simulink model "sim_model_ss"  (R2018b)
settings: Solver=VariableStepAuto  StartTime=0.0  StopTime=10.0  RelTol=1e-3
values from neighbouring files (symbols this model uses):
  A = J    [Main.m]
  B = [0;0;K6]    [Main.m]
  C1 = [1, 0, 0]    [Main.m]
  C2 = [0, 1, 0]    [Main.m]
  C3 = [0, 0, 1]    [Main.m]
  D = 0    [Main.m]
  u0 = er    [Main.m]
  x10 = 0.03    [Main.m]
  x20 = v0    (= 0)    [Main.m]
  x30 = I0    [Main.m]
settings Model: Creator=Eduardo  LastModifiedBy=ohara

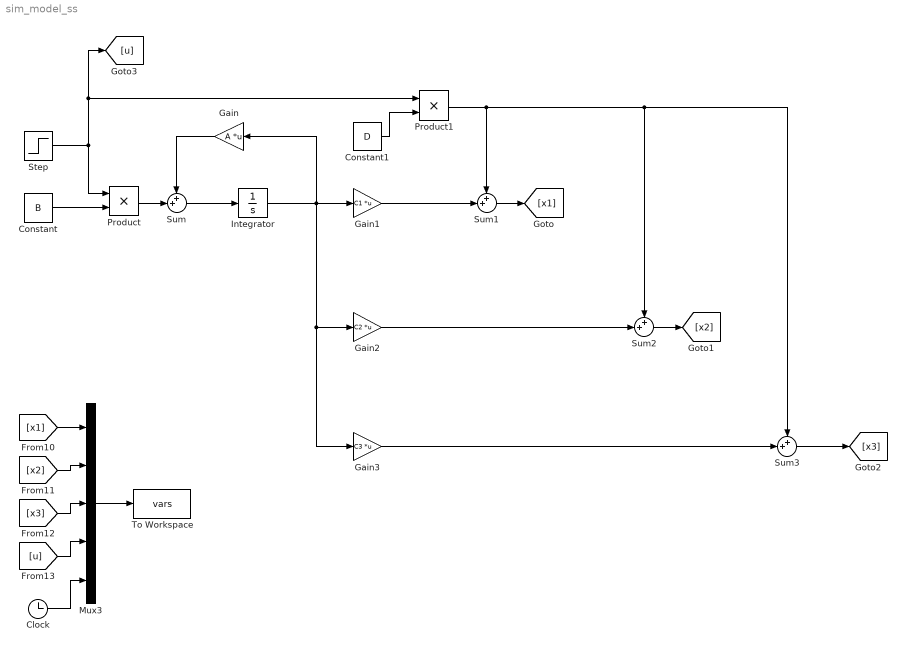
== system sim_model_ss ==
  Clock : Clock
  Constant : Constant  Value=B
  Constant1 : Constant  Value=D
  Gain : Gain  Gain=A  Multiplication=Matrix(K*u)
  Gain1 : Gain  Gain=C1  Multiplication=Matrix(K*u)
  Gain2 : Gain  Gain=C2  Multiplication=Matrix(K*u)
  Gain3 : Gain  Gain=C3  Multiplication=Matrix(K*u)
  Integrator : Integrator  InitialCondition=[x10;x20;x30]
  Mux3 : Mux  Inputs=5
  Product : Product
  Product1 : Product
  Step : Step  Time=0  Before=u0  After=u0  SampleTime=0
  Sum{,1..3} (4 alike) : Sum  Inputs=++|
  To Workspace : ToWorkspace  VariableName=vars  SaveFormat=Timeseries  SampleTime=-1
  wires:
  Sum/1 -> Integrator/1
  Product/1 -> Sum/2
  Constant/1 -> Product/2
  Step/1 -> Product/1, [u], Product1/1
  Gain/1 -> Sum/1
  Integrator/1 -> Gain2/1, Gain3/1, Gain1/1, Gain/1
  Gain1/1 -> Sum1/2
  Product1/1 -> Sum2/1, Sum3/1, Sum1/1
  Constant1/1 -> Product1/2
  Sum1/1 -> [x1]
  Gain2/1 -> Sum2/2
  Sum2/1 -> [x2]
  Gain3/1 -> Sum3/2
  Sum3/1 -> [x3]
  [x1] -> Mux3/1
  Clock/1 -> Mux3/5
  Mux3/1 -> To Workspace/1
  [x3] -> Mux3/3
  [u] -> Mux3/4
  [x2] -> Mux3/2
